simulink model "sensores_ideales"  (R2023b)
settings: Solver=VariableStepAuto  StartTime=0.0  StopTime=10.0  RelTol=1e-3
settings Model: Creator=Pc  LastModifiedBy=Pc

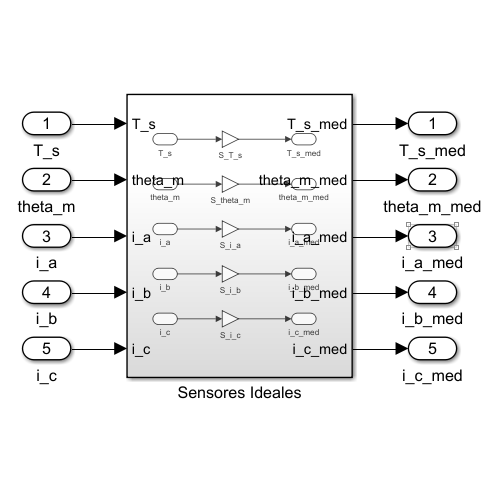
[thumbnail: Simulink's stored preview of the top-level diagram]
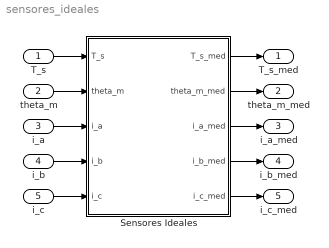
== system sensores_ideales ==
  T_s : Inport
  theta_m : Inport  Port=2
  i_a : Inport  Port=3
  i_b : Inport  Port=4
  i_c : Inport  Port=5
  Sensores Ideales : Subsystem
  T_s_med : Outport
  theta_m_med : Outport  Port=2
  i_a_med : Outport  Port=3
  i_b_med : Outport  Port=4
  i_c_med : Outport  Port=5
  wires:
  T_s/1 -> Sensores Ideales/1(T_s)
  theta_m/1 -> Sensores Ideales/2(theta_m)
  i_a/1 -> Sensores Ideales/3(i_a)
  i_b/1 -> Sensores Ideales/4(i_b)
  i_c/1 -> Sensores Ideales/5(i_c)
  Sensores Ideales/1(T_s_med) -> T_s_med/1
  Sensores Ideales/2(theta_m_med) -> theta_m_med/1
  Sensores Ideales/3(i_a_med) -> i_a_med/1
  Sensores Ideales/4(i_b_med) -> i_b_med/1
  Sensores Ideales/5(i_c_med) -> i_c_med/1

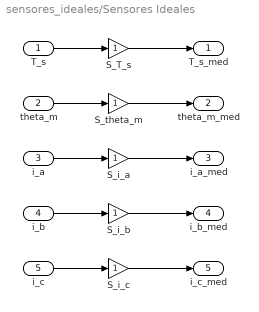
== system sensores_ideales/Sensores Ideales ==
  T_s : Inport
  theta_m : Inport  Port=2
  i_a : Inport  Port=3
  i_b : Inport  Port=4
  i_c : Inport  Port=5
  S_T_s : Gain
  S_i_a : Gain
  S_i_b : Gain
  S_i_c : Gain
  S_theta_m : Gain
  T_s_med : Outport
  theta_m_med : Outport  Port=2
  i_a_med : Outport  Port=3
  i_b_med : Outport  Port=4
  i_c_med : Outport  Port=5
  wires:
  i_a/1 -> S_i_a/1
  T_s/1 -> S_T_s/1
  S_theta_m/1 -> theta_m_med/1
  theta_m/1 -> S_theta_m/1
  S_i_c/1 -> i_c_med/1
  i_b/1 -> S_i_b/1
  i_c/1 -> S_i_c/1
  S_T_s/1 -> T_s_med/1
  S_i_b/1 -> i_b_med/1
  S_i_a/1 -> i_a_med/1
